simulink model "SolarDCACInverter"  (R2021a)
settings: Solver=VariableStepAuto  StartTime=0.0  StopTime=1  RelTol=1e-3
libraries: spsSeriesRLCBranchLib x13, spsIGBTDiodeLib x6, spsCurrentMeasurementLib x3, simulink x3, spsVoltageMeasurementLib x3, spsGroundLib x1, spsPVArrayLib x1, spspowerguiLib x1
settings Model: Creator=Nilay Mundra  LastModifiedBy=Nilay Mundra

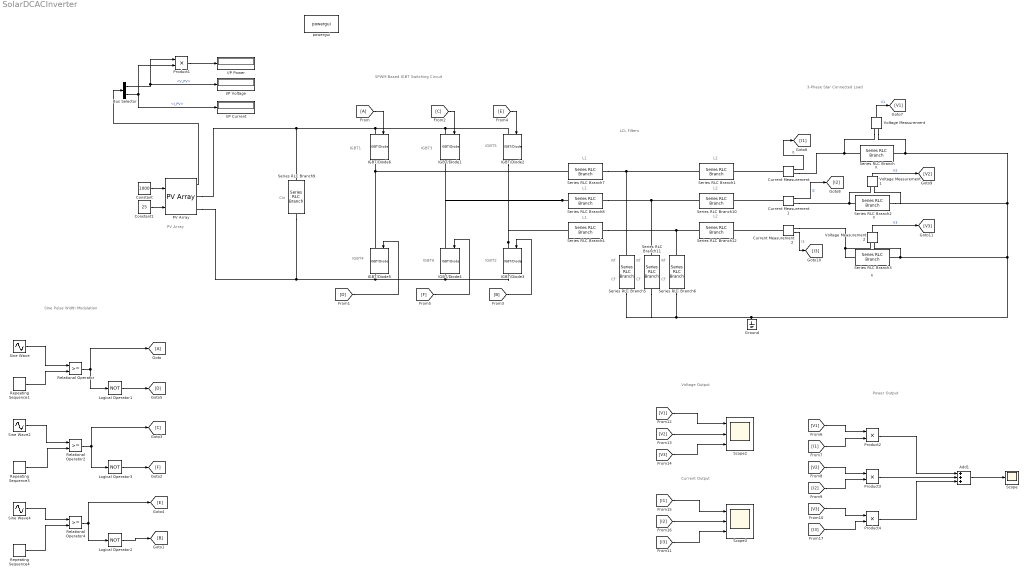
== system SolarDCACInverter ==
  note: LCL Filters
  note: Power Output
  note: IGBT2
  note: IGBT4
  note: IGBT3
  note: IGBT5
  note: IGBT6
  note: IGBT1
  note: Voltage Output
  note: Current Output
  note: 3-Phase Star Connected Load
  note: PV Array
  note: SPWM Based IGBT Switching Circuit
  note: SIne Pulse Width Modulation
  note: Cin
  note: L1
  note: L1
  note: L1
  note: L2
  note: L2
  note: L2
  note: Rf
  note: Rf
  note: Rf
  note: Cf
  note: Cf
  note: Cf
  note: R
  note: R
  note: R
  Add1 : Sum  Inputs=+++
  Bus Selector : BusSelector  OutputSignals=V_PV,I_PV
  Constant : Constant  Value=1000
  Constant1 : Constant  Value=25
  Current Measurement : spsCurrentMeasurementLib/Current Measurement  PhasorSimulation=off  OutputType=Complex  PSBequivalent=0
  Current Measurement1 : spsCurrentMeasurementLib/Current Measurement  PhasorSimulation=off  OutputType=Complex  PSBequivalent=0
  Current Measurement2 : spsCurrentMeasurementLib/Current Measurement  PhasorSimulation=off  OutputType=Complex  PSBequivalent=0
  Ground : spsGroundLib/Ground  LConnTagsString=a
  I/P Current : Display
  I/P Power : Display
  I/P Voltage : Display
  IGBT/Diode{1..6} (6 alike) : spsIGBTDiodeLib/IGBT//Diode  Ron=1e-3  Rs=1e5  Cs=inf  Measurements=on
  Logical Operator1 : Logic  Operator=NOT  AllPortsSameDT=off  OutDataTypeStr=boolean
  Logical Operator2 : Logic  Operator=NOT  AllPortsSameDT=off  OutDataTypeStr=boolean
  Logical Operator3 : Logic  Operator=NOT  AllPortsSameDT=off  OutDataTypeStr=boolean
  PV Array : spsPVArrayLib/PV Array  Npar=1  Nser=1  PlotType=array @ 1000 W/m2 & specified temperatures  S_vec="[ 1000  500  100 ]"  Temp_C_vec="[ 45 25  ]"  ModuleName=A10Green Technology A10J-S72-175  PlotWhenSelected=off  Pm=175.0914  Ncell=72  Voc=43.99  Isc=5.17  Vm=36.63  Im=4.78  beta_Voc_pc=-0.3616  alpha_Isc_pc=0.041509  beta_Voc=-0.15907  alpha_Isc=0.002146  IL=5.178  I0=1.7842e-10  nI=0.98852  Rsh=249.6758  Rs=0.38412  RobustModel=off  RobustCellTemperature=313.3991  BAL=on  Tc=1e-6  Tfilter=5e-5
  Product{1..4} (4 alike) : Product
  Relational Operator : RelationalOperator  OutDataTypeStr=boolean  RndMeth=Simplest
  Relational Operator2 : RelationalOperator  OutDataTypeStr=boolean  RndMeth=Simplest
  Relational Operator4 : RelationalOperator  OutDataTypeStr=boolean  RndMeth=Simplest
  Repeating Sequence1 : simulink/Sources/Repeating Sequence  rep_seq_t=[0 1 2 3 4] * (1/20000)  rep_seq_y=[0 1 0 -1 0]
  Repeating Sequence3 : simulink/Sources/Repeating Sequence  rep_seq_t=[0 1 2 3 4] * (1/20000)  rep_seq_y=[0 1 0 -1 0]
  Repeating Sequence4 : simulink/Sources/Repeating Sequence  rep_seq_t=[0 1 2 3 4] * (1/20000)  rep_seq_y=[0 1 0 -1 0]
  Scope : Scope
  Scope2 : Scope  NumInputPorts=3
  Scope3 : Scope  NumInputPorts=3
  Series RLC Branch : spsSeriesRLCBranchLib/Series RLC Branch  LConnTagsString=__new0  RConnTagsString=__new0  BranchType=R  Resistance=1.84  Inductance=1e-3  SetiL0=off  InitialCurrent=0  Capacitance=1e-6  Setx0=off  InitialVoltage=0  Measurements=None
  Series RLC Branch1 : spsSeriesRLCBranchLib/Series RLC Branch  LConnTagsString=__new0  RConnTagsString=__new0  BranchType=L  Resistance=1  Inductance=7.0251e-05  SetiL0=off  InitialCurrent=0  Capacitance=1e-6  Setx0=off  InitialVoltage=0  Measurements=None
  Series RLC Branch10 : spsSeriesRLCBranchLib/Series RLC Branch  LConnTagsString=__new0  RConnTagsString=__new0  BranchType=L  Resistance=1  Inductance=7.0251e-05  SetiL0=off  InitialCurrent=0  Capacitance=1e-6  Setx0=off  InitialVoltage=0  Measurements=None
  Series RLC Branch11 : spsSeriesRLCBranchLib/Series RLC Branch  LConnTagsString=__new0  RConnTagsString=__new0  BranchType=RC  Resistance=0.2937  Inductance=1e-3  SetiL0=off  InitialCurrent=0  Capacitance=8.6537e-05  Setx0=off  InitialVoltage=0  Measurements=None
  Series RLC Branch12 : spsSeriesRLCBranchLib/Series RLC Branch  LConnTagsString=__new0  RConnTagsString=__new0  BranchType=L  Resistance=1  Inductance=7.0251e-05  SetiL0=off  InitialCurrent=0  Capacitance=1e-6  Setx0=off  InitialVoltage=0  Measurements=None
  Series RLC Branch2 : spsSeriesRLCBranchLib/Series RLC Branch  LConnTagsString=__new0  RConnTagsString=__new0  BranchType=R  Resistance=1.84  Inductance=1e-3  SetiL0=off  InitialCurrent=0  Capacitance=1e-6  Setx0=off  InitialVoltage=0  Measurements=None
  Series RLC Branch3 : spsSeriesRLCBranchLib/Series RLC Branch  LConnTagsString=__new0  RConnTagsString=__new0  BranchType=R  Resistance=1.84  Inductance=1e-3  SetiL0=off  InitialCurrent=0  Capacitance=1e-6  Setx0=off  InitialVoltage=0  Measurements=None
  Series RLC Branch4 : spsSeriesRLCBranchLib/Series RLC Branch  LConnTagsString=__new0  RConnTagsString=__new0  BranchType=L  Resistance=1  Inductance=1.5e-3  SetiL0=off  InitialCurrent=0  Capacitance=1e-6  Setx0=off  InitialVoltage=0  Measurements=None
  Series RLC Branch5 : spsSeriesRLCBranchLib/Series RLC Branch  LConnTagsString=__new0  RConnTagsString=__new0  BranchType=RC  Resistance=0.2937  Inductance=1e-3  SetiL0=off  InitialCurrent=0  Capacitance=8.6537e-05  Setx0=off  InitialVoltage=0  Measurements=None
  Series RLC Branch6 : spsSeriesRLCBranchLib/Series RLC Branch  LConnTagsString=__new0  RConnTagsString=__new0  BranchType=RC  Resistance=0.2937  Inductance=1e-3  SetiL0=off  InitialCurrent=0  Capacitance=8.6537e-05  Setx0=off  InitialVoltage=0  Measurements=None
  Series RLC Branch7 : spsSeriesRLCBranchLib/Series RLC Branch  LConnTagsString=__new0  RConnTagsString=__new0  BranchType=L  Resistance=1  Inductance=1.5e-3  SetiL0=off  InitialCurrent=0  Capacitance=1e-6  Setx0=off  InitialVoltage=0  Measurements=None
  Series RLC Branch8 : spsSeriesRLCBranchLib/Series RLC Branch  LConnTagsString=__new0  RConnTagsString=__new0  BranchType=L  Resistance=1  Inductance=1.5e-3  SetiL0=off  InitialCurrent=0  Capacitance=1e-6  Setx0=off  InitialVoltage=0  Measurements=None
  Series RLC Branch9 : spsSeriesRLCBranchLib/Series RLC Branch  LConnTagsString=__new0  RConnTagsString=__new0  BranchType=C  Resistance=1  Inductance=1e-3  SetiL0=off  InitialCurrent=0  Capacitance=0.01  Setx0=off  InitialVoltage=36.3  Measurements=None
  Sine Wave : Sin  Amplitude=0.8  Frequency=314  SampleTime=0
  Sine Wave2 : Sin  Amplitude=0.8  Frequency=314  Phase=2*pi/3  SampleTime=0
  Sine Wave4 : Sin  Amplitude=0.8  Frequency=314  Phase=4*pi/3  SampleTime=0
  Voltage Measurement : spsVoltageMeasurementLib/Voltage Measurement  PhasorSimulation=off  OutputType=Complex  PSBequivalent=0
  Voltage Measurement1 : spsVoltageMeasurementLib/Voltage Measurement  PhasorSimulation=off  OutputType=Complex  PSBequivalent=0
  Voltage Measurement2 : spsVoltageMeasurementLib/Voltage Measurement  PhasorSimulation=off  OutputType=Complex  PSBequivalent=0
  powergui : spspowerguiLib/powergui  Priority=1  SimulationMode=Discrete  SampleTime=50e-7  frequency=60  Iterations=50  frequencyindice=0  Pbase=100e6  ErrMax=1e-4  UnitsV=kV  UnitsW=MW  buscounter=0  FunctionMessages=off  echomessages=off  EnableUseOfTLC=off  CurrentSourceSwitches=off  DisableSnubberDevices=off  DisableRonSwitches=off  DisableVfSwitches=off  DisplayEquations=off  AutomaticDiscreteSolvers=off  SolverType=Tustin/Backward Euler (TBE)  Interpol=off  ExternalGateDelay=off  methode=off  Ts=100  x0status=blocks  SPID=on  SwTol=0  HookPort=off  NonlinearTolerance=1e-4  nMaxIteration=100  ContinueOnMaxIteration=off  RestoreLinks=warning  ResistiveCurrentMeasurement=off  Frange=[0:2:500]  Ylog=off  Xlog=on  ShowGrid=off  save=off  variable=ZData  structure=0  ZoomFFT=off  StartTime=0.0  cycles=1  DisplayStyle=1  fundamental=60  FreqAxis=off  MaxFrequency=1000  frequencyindicesteady=1  RmsSteady=1  display=off
  wires:
  Relational Operator4/1 -> Logical Operator2/1, [E]
  Sine Wave4/1 -> Relational Operator4/1
  Sine Wave2/1 -> Relational Operator2/1
  [F] -> IGBT/Diode4/1
  [C] -> IGBT/Diode1/1
  [D] -> IGBT/Diode5/1
  Relational Operator/1 -> Logical Operator1/1, [A]
  [B] -> IGBT/Diode3/1
  [E] -> IGBT/Diode2/1
  [A] -> IGBT/Diode6/1
  Repeating Sequence1/1 -> Relational Operator/2
  Repeating Sequence3/1 -> Relational Operator2/2
  Repeating Sequence4/1 -> Relational Operator4/2
  Sine Wave/1 -> Relational Operator/1
  Constant1/1 -> PV Array/2
  Constant/1 -> PV Array/1
  Bus Selector/2 -> Product1/2, I/P Current/1  "<I_PV>"
  Bus Selector/1 -> Product1/1, I/P Voltage/1  "<V_PV>"
  Product1/1 -> I/P Power/1
  PV Array/1 -> Bus Selector/1
  Logical Operator2/1 -> [B]
  Relational Operator2/1 -> [C], Logical Operator3/1
  Logical Operator1/1 -> [D]
  Logical Operator3/1 -> [F]
  Current Measurement/1 -> [I1]  "I1"
  Voltage Measurement/1 -> [V1]  "V1"
  Voltage Measurement1/1 -> [V2]  "V2"
  Voltage Measurement2/1 -> [V3]  "V3"
  Current Measurement1/1 -> [I2]  "I2"
  Current Measurement2/1 -> [I3]  "I3"
  [V1] -> Product2/1
  [I1] -> Product2/2
  [V2] -> Product3/1
  [I2] -> Product3/2
  [V3] -> Product4/1
  [I3] -> Product4/2
  Product2/1 -> Add1/1
  Product3/1 -> Add1/2
  Product4/1 -> Add1/3
  Add1/1 -> Scope/1
  [V1] -> Scope2/1
  [V2] -> Scope2/2
  [V3] -> Scope2/3
  [I2] -> Scope3/2
  [I1] -> Scope3/1
  [I3] -> Scope3/3
  connections:
  Series RLC Branch9/LConn1 -- IGBT/Diode6/LConn1 -- IGBT/Diode1/LConn1 -- IGBT/Diode2/LConn1 -- PV Array/RConn1
  IGBT/Diode3/LConn1 -- IGBT/Diode2/RConn1 -- Series RLC Branch4/LConn1
  Series RLC Branch9/RConn1 -- IGBT/Diode5/RConn1 -- IGBT/Diode3/RConn1 -- IGBT/Diode4/RConn1 -- PV Array/RConn2
  Current Measurement/RConn1 -- Voltage Measurement/LConn1 -- Series RLC Branch/LConn1
  IGBT/Diode5/LConn1 -- Series RLC Branch7/LConn1 -- IGBT/Diode6/RConn1
  Series RLC Branch7/RConn1 -- Series RLC Branch5/LConn1 -- Series RLC Branch1/LConn1
  Current Measurement2/LConn1 -- Series RLC Branch12/RConn1
  Series RLC Branch8/LConn1 -- IGBT/Diode4/LConn1 -- IGBT/Diode1/RConn1
  Current Measurement/LConn1 -- Series RLC Branch1/RConn1
  Series RLC Branch8/RConn1 -- Series RLC Branch11/LConn1 -- Series RLC Branch10/LConn1
  Series RLC Branch4/RConn1 -- Series RLC Branch6/LConn1 -- Series RLC Branch12/LConn1
  Voltage Measurement/LConn2 -- Voltage Measurement1/LConn2 -- Series RLC Branch2/RConn1 -- Series RLC Branch5/RConn1 -- Series RLC Branch11/RConn1 -- Series RLC Branch6/RConn1 -- Ground/LConn1 -- Voltage Measurement2/LConn2 -- Series RLC Branch3/RConn1 -- Series RLC Branch/RConn1
  Current Measurement1/LConn1 -- Series RLC Branch10/RConn1
  Current Measurement1/RConn1 -- Voltage Measurement1/LConn1 -- Series RLC Branch2/LConn1
  Current Measurement2/RConn1 -- Voltage Measurement2/LConn1 -- Series RLC Branch3/LConn1
